simulink model "resp"  (R2021a)
settings: Solver=VariableStepAuto  StartTime=0.0  StopTime=10.0  RelTol=1e-3
values from neighbouring files (symbols this model uses):
  j = str2num(get(handles.Rp, 'String'))    [Ventiladorcito.m]
settings Model: Creator=sajit  LastModifiedBy=sajit

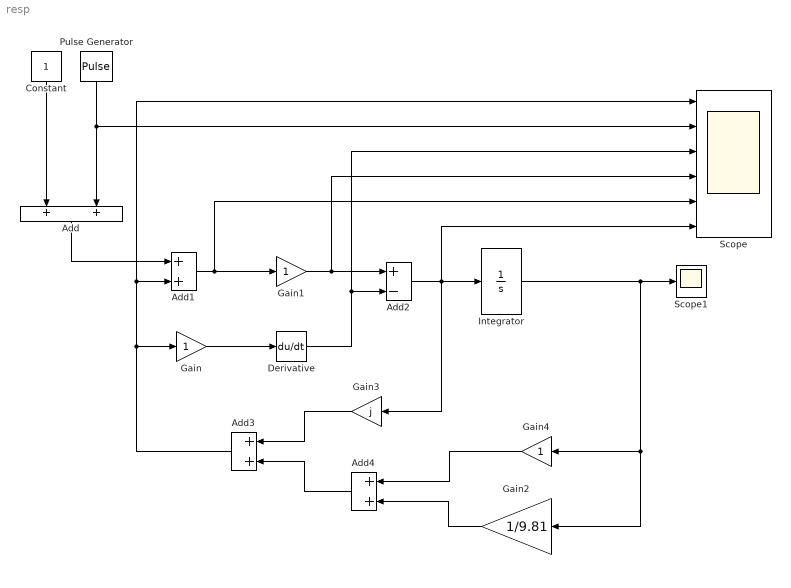
== system resp ==
  Add{,1,3..4} (4 alike) : Sum
  Add2 : Sum  Inputs=+-
  Constant : Constant
  Derivative : Derivative
  Gain : Gain
  Gain1 : Gain
  Gain2 : Gain  Gain=1/9.81
  Gain3 : Gain  Gain=j
  Gain4 : Gain
  Integrator : Integrator  InitialCondition=0.1
  Pulse Generator : DiscretePulseGenerator  PulseType=Time based  Period=10  PulseWidth=5
  Scope : Scope  NumInputPorts=6
  Scope1 : Scope
  wires:
  Pulse Generator/1 -> Add/2, Scope/2
  Add/1 -> Add1/1
  Add1/1 -> Scope/5, Gain1/1
  Gain1/1 -> Scope/4, Add2/1
  Derivative/1 -> Scope/3, Add2/2
  Gain/1 -> Derivative/1
  Add3/1 -> Gain/1, Scope/1, Add1/2
  Gain4/1 -> Add4/1
  Gain2/1 -> Add4/2
  Add4/1 -> Add3/2
  Gain3/1 -> Add3/1
  Add2/1 -> Scope/6, Gain3/1, Integrator/1
  Integrator/1 -> Gain2/1, Gain4/1, Scope1/1
  Constant/1 -> Add/1
